simulink model "uz_pmsm_rfe"  (R2023a)
settings: Solver=FixedStepDiscrete  StartTime=0.0  StopTime=50  RelTol=1e-3  EnableMultiTasking=on
PreLoadFcn:
  | uz_setCodegenPaths
model workspace (MATLAB code in the model file):
  | cmdLim = Simulink.Parameter;
  | cmdLim.Value = 15;
  | cmdLim.Description = 'Limit for controlling the maximum surface command angle.';
  | cmdLim.Min = 0;
  | cmdLim.Max = 90;
  | cmdLim.DocUnits = 'deg';
  | 
  | dispGain = Simulink.Parameter;
  | dispGain.Value = 0.75;
  | dispGain.Description = 'Gain applied to the displacement error.';
  | dispGain.Min = 0;
  | dispGain.Max = [];
  | dispGain.DocUnits = 'deg/sec/deg';
  | 
  | dispLim = Simulink.Parameter;
  | dispLim.Value = 30;
  | dispLim.Description = 'Limit for controlling the maximum commanded angle.';
  | dispLim.Min = 0;
  | dispLim.Max = 180;
  | dispLim.DocUnits = 'deg';
  | 
  | intGain = Simulink.Parameter;
  | intGain.Value = 0.5;
  | intGain.Description = 'Gain applied to the integral error.';
  | intGain.Min = 0;
  | intGain.Max = [];
  | intGain.DocUnits = 'deg/sec/deg/sec';
  | 
  | intLim = Simulink.Parameter;
  | intLim.Value = 5;
  | intLim.Description = 'Limit for controlling the maximum commanded angle.';
  | intLim.Min = 0;
  | intLim.Max = 90;
  | intLim.DocUnits = 'deg';
  | 
  | rateGain = Simulink.Parameter;
  | rateGain.Value = 2;
  | rateGain.Description = 'Gain applied to the rate error.';
  | rateGain.Min = 0;
  | rateGain.Max = [];
  | rateGain.DocUnits = 'deg/deg/sec';
  | 
  | rateLim = Simulink.Parameter;
  | rateLim.Value = 6;
  | rateLim.Description = 'Limit for controlling the maximum commanded angle.';
  | rateLim.Min = 0;
  | rateLim.Max = 180;
  | rateLim.DocUnits = 'deg/sec';
  | 
  | hdgGain = Simulink.Parameter;
  | hdgGain.Value = 0.015;
undefined symbols (not defined in the file): DiscIntNeverNeededParam, Ld, Lq, PN, psi_pm, r_cd, r_cq, r_s
settings Model: RequirementInfo={} %GIDa_fe9045fd_0412_4b6e_8206_617cc20e6fde  Creator=ts  LastModifiedBy=ts
settings SolverCC: AlgebraicLoopSolver=TrustRegion  PositivePriorityOrder=on  AutoInsertRateTranBlk=on
settings DataIOCC: SaveOutput=off  SignalLogging=off  DSMLogging=off  SaveTime=off
settings OptimizationCC: DefaultParameterBehavior=Inlined  UseDivisionForNetSlopeComputation=on  GainParamInheritBuiltInType=on  UseFloatMulNetSlope=on  UseSpecifiedMinMax=on  InlineInvariantSignals=on  PassReuseOutputArgsAs=Individual arguments  NoFixptDivByZeroProtection=on  EfficientFloat2IntCast=on  LifeSpan=1  MaxStackSize=64  OptimizeBlockOrder=speed  DifferentSizesBufferReuse=on  EfficientTunableParamExpr=on
settings DebuggingCC: UnconnectedInputMsg=warning  UnconnectedOutputMsg=warning  UnconnectedLineMsg=warning  AllowSymbolicDim=off  SFUnexpectedBacktrackingDiag=warning  SFNoUnconditionalDefaultTransitionDiag=warning  SFExecutionAtInitializationDiag=none  ArithmeticOperatorsInVariantConditions=warning
settings HardwareCC: ProdBitPerPointer=32  ProdBitPerSizeT=32  ProdBitPerPtrDiffT=32  ProdLargestAtomicInteger=Long  ProdLargestAtomicFloat=Double  ProdWordSize=32  ProdLongLongMode=on  ProdHWDeviceType=ARM Compatible->ARM Cortex-R  HardwareBoardFeatureSet=SoCBlockset
settings ModelReferenceCC: EnableRefExpFcnMdlSchedulingChecks=on
settings SFSimCC: MATLABDynamicMemAlloc=off
settings RTWCC: Description=Embedded Coder  SystemTargetFile=ert.tlc  GenCodeOnly=on  TemplateMakefile=ert_default_tmf  GenerateReport=on  BuildConfiguration=Faster Runs  IncludeHyperlinkInReport=on  GenerateCodeMetricsReport=on  CheckMdlBeforeBuild=Warning  DLArmComputeVersion=19.05
settings CodeAppCC: ForceParamTrailComments=on  IgnoreCustomStorageClasses=off  OperatorAnnotations=on  SimulinkDataObjDesc=on  SFDataObjDesc=on  MATLABFcnDesc=on  CustomSymbolStrGlobalVar=rt$N$M  CustomSymbolStrType=$N$M  CustomSymbolStrFcn=$N$M$F  CustomSymbolStrMacro=$N$M  InsertBlockDesc=on  StateflowObjectComments=on  MATLABSourceComments=on  EnableCustomComments=on  ReqsInCode=on
settings ERTTargetCC: TargetLangStandard=C99 (ISO)  CodeReplacementLibrary=GNU C99 extensions  MultiwordLength=2048  IncludeMdlTerminateFcn=off  CombineSignalStateStructs=on  SuppressErrorStatus=on  IncludeFileDelimiter=UseQuote  SupportAbsoluteTime=off  CodeInterfacePackaging=Reusable function  SupportNonFinite=off  RemoveResetFunc=off  InlinedParameterPlacement=NonHierarchical  MultiInstanceErrorCode=Warning  RootIOFormat=Part of model data structure  ERTCustomFileTemplate=example_file_process.tlc  GlobalDataDefinition=InSourceFile  GlobalDataReference=InSourceFile  ERTFilePackagingFormat=CompactWithDataFile
settings ConfigComp: CovScope=ReferencedModels  CovSaveName=covdata_rollAP  CovMetricSettings=dcmtrwe  CovHTMLOptions=-sRT=1 -aTS=1 -bRG=1 -bTC=1 -hTR=1 -nFC=0 -scm=1 -bcm=1 -xEv=0  CovSaveCumulativeToWorkspaceVar=on  CovSaveSingleToWorkspaceVar=on  CovCumulativeVarName=covCumulativeData_rollAP  CovReportOnPause=off  CovExternalEMLEnable=off  CovSFcnEnable=off

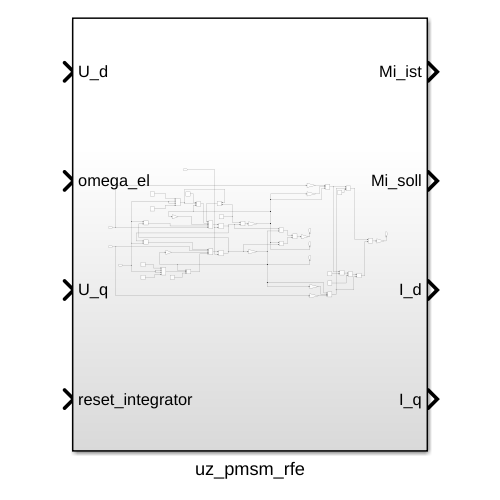
[thumbnail: Simulink's stored preview of the top-level diagram]
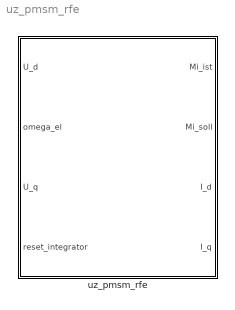
== system uz_pmsm_rfe ==
  uz_pmsm_rfe : Subsystem

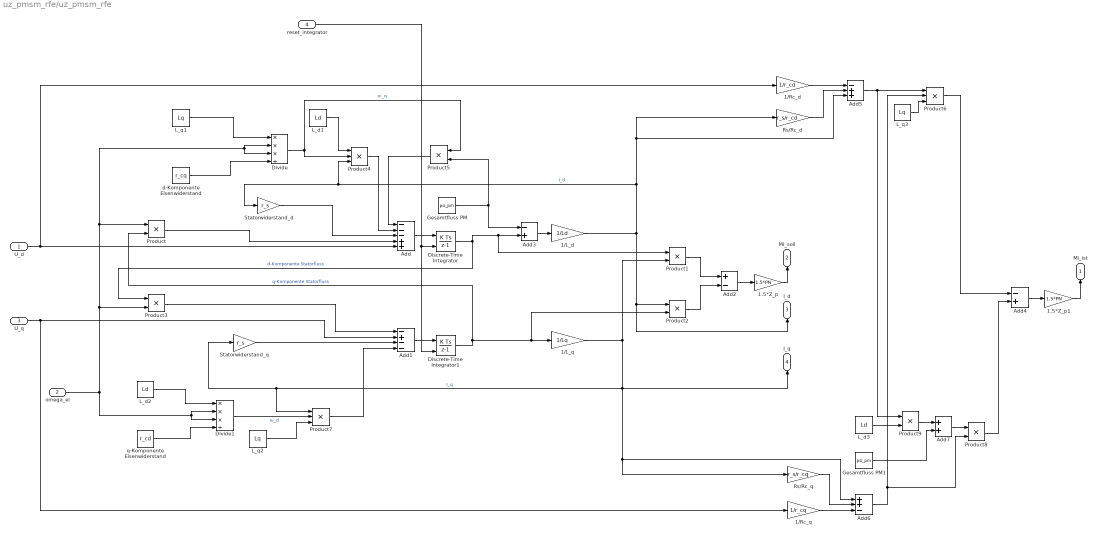
== system uz_pmsm_rfe/uz_pmsm_rfe ==
  U_d : Inport
  omega_el : Inport  Port=2
  U_q : Inport  Port=3
  reset_integrator : Inport  Port=4
  1.5*Z_p : Gain  Gain=1.5*PN
  1.5*Z_p1 : Gain  Gain=1.5*PN
  1/L_d : Gain  Gain=1/Ld
  1/L_q : Gain  Gain=1/Lq
  1/Rc_d : Gain  Gain=1/r_cd
  1/Rc_q : Gain  Gain=1/r_cq
  Add : Sum  Inputs=---++
  Add1 : Sum  Inputs=-+--
  Add2 : Sum  Inputs=+-
  Add3 : Sum  Inputs=-+
  Add4 : Sum  Inputs=-+
  Add5 : Sum  Inputs=-++
  Add6 : Sum  Inputs=++-
  Add7 : Sum
  Discrete-Time Integrator : DiscreteIntegrator  ExternalReset=rising  SampleTime=-1  ICPrevOutput=DiscIntNeverNeededParam  ICPrevScaledInput=DiscIntNeverNeededParam
  Discrete-Time Integrator1 : DiscreteIntegrator  ExternalReset=rising  SampleTime=-1  ICPrevOutput=DiscIntNeverNeededParam  ICPrevScaledInput=DiscIntNeverNeededParam
  Divide : Product  Inputs=***/
  Divide1 : Product  Inputs=***/
  Gesamtfluss PM : Constant  Value=psi_pm
  Gesamtfluss PM1 : Constant  Value=psi_pm
  L_d1 : Constant  Value=Ld
  L_d2 : Constant  Value=Ld
  L_d3 : Constant  Value=Ld
  L_q1 : Constant  Value=Lq
  L_q2 : Constant  Value=Lq
  L_q3 : Constant  Value=Lq
  Product{,1..3,5,8..9} (7 alike) : Product
  Product4 : Product  Inputs=3
  Product6 : Product  Inputs=3
  Product7 : Product  Inputs=3
  Rs/Rc_d : Gain  Gain=r_s/r_cd
  Rs/Rc_q : Gain  Gain=r_s/r_cq
  Statorwiderstand_d : Gain  Gain=r_s
  Statorwiderstand_q : Gain  Gain=r_s
  d-Komponente Eisenwiderstand : Constant  Value=r_cq
  q-Komponente Eisenwiderstand : Constant  Value=r_cd
  Mi_ist : Outport
  Mi_soll : Outport  Port=2
  I_d : Outport  Port=3
  I_q : Outport  Port=4
  wires:
  omega_el/1 -> Product3/2, Product/1, Divide/3, Divide/2, Divide1/2, Divide1/3
  Product/1 -> Add/4
  d-Komponente Eisenwiderstand/1 -> Divide/4
  Gesamtfluss PM/1 -> Product5/2, Add3/1
  Add5/1 -> Product9/1, Product6/1
  1.5*Z_p/1 -> Mi_soll/1
  Product3/1 -> Add1/1
  1/L_q/1 -> Product1/2, Statorwiderstand_q/1, Product7/1, Rs/Rc_q/1, Add6/1, I_q/1  "I_q"
  Divide1/1 -> Product7/2  "xi_d"
  Add2/1 -> 1.5*Z_p/1
  L_q1/1 -> Divide/1
  Product7/1 -> Add1/4
  Divide/1 -> Product4/2, Product5/1  "xi_q"
  Statorwiderstand_d/1 -> Add/3
  Product4/1 -> Add/2
  Rs/Rc_q/1 -> Add6/2
  Product5/1 -> Add/1
  1/L_d/1 -> Product4/3, Statorwiderstand_d/1, Rs/Rc_d/1, Add5/3, I_d/1, Product2/1  "I_d"
  Product2/1 -> Add2/2
  Product1/1 -> Add2/1
  Add1/1 -> Discrete-Time Integrator1/1
  Add/1 -> Discrete-Time Integrator/1
  Product6/1 -> Add4/1
  q-Komponente Eisenwiderstand/1 -> Divide1/4
  Add6/1 -> Product8/2, Product6/2
  Statorwiderstand_q/1 -> Add1/3
  reset_integrator/1 -> Discrete-Time Integrator1/2, Discrete-Time Integrator/2
  1/Rc_q/1 -> Add6/3
  Discrete-Time Integrator/1 -> Add3/2, Product1/1, Product3/1  "d-Komponente Statorfluss"
  L_d1/1 -> Product4/1
  Add3/1 -> 1/L_d/1
  U_d/1 -> Add/5, 1/Rc_d/1
  1/Rc_d/1 -> Add5/1
  L_q3/1 -> Product6/3
  Add4/1 -> 1.5*Z_p1/1
  Rs/Rc_d/1 -> Add5/2
  L_d2/1 -> Divide1/1
  1.5*Z_p1/1 -> Mi_ist/1
  L_q2/1 -> Product7/3
  Product8/1 -> Add4/2
  L_d3/1 -> Product9/2
  Gesamtfluss PM1/1 -> Add7/2
  U_q/1 -> 1/Rc_q/1, Add1/2
  Product9/1 -> Add7/1
  Add7/1 -> Product8/1
  Discrete-Time Integrator1/1 -> Product/2, Product2/2, 1/L_q/1  "q-Komponente Statorfluss"
